simulink model "SDT505SimpleMotorModelBatteryModule220119"  (R2022b)
settings: Solver=VariableStepAuto  StartTime=0.0  StopTime=10.0  RelTol=1e-3
settings Model: Creator=mjbou  LastModifiedBy=mjbou
settings SolverCC: AlgebraicLoopSolver=TrustRegion
settings DebuggingCC: UnconnectedInputMsg=warning  UnconnectedOutputMsg=warning  UnconnectedLineMsg=warning  SFMachineParentedDataDiag=warning
settings ModelReferenceCC: EnableRefExpFcnMdlSchedulingChecks=on

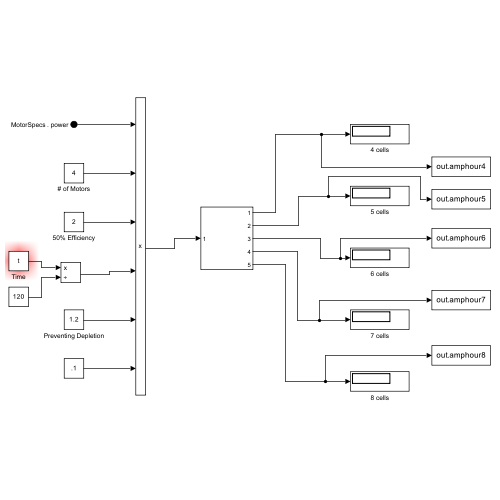
[thumbnail: Simulink's stored preview of the top-level diagram]
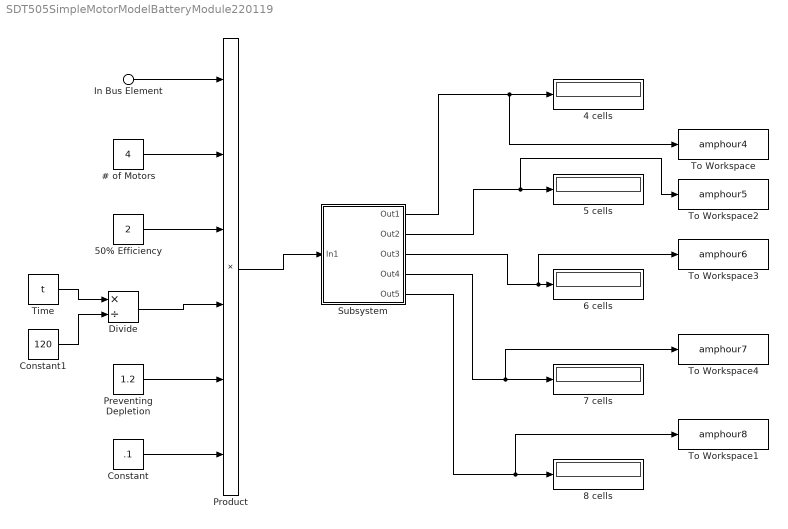
== system SDT505SimpleMotorModelBatteryModule220119 ==
  In Bus Element : Inport  PortName=MotorSpecs  Element=power
  # of Motors : Constant  Value=4
  4 cells : Display
  5 cells : Display
  50% Efficiency : Constant  Value=2
  6 cells : Display
  7 cells : Display
  8 cells : Display
  Constant : Constant  Value=.1
  Constant1 : Constant  Value=120
  Divide : Product  Inputs=*/
  Preventing Depletion : Constant  Value=1.2
  Product : Product  Inputs=6
  Subsystem : Subsystem
  Time : Constant  Value=t
  To Workspace : ToWorkspace  VariableName=amphour4  SaveFormat=Timeseries  SampleTime=-1
  To Workspace1 : ToWorkspace  VariableName=amphour8  SaveFormat=Timeseries  SampleTime=-1
  To Workspace2 : ToWorkspace  VariableName=amphour5  SaveFormat=Timeseries  SampleTime=-1
  To Workspace3 : ToWorkspace  VariableName=amphour6  SaveFormat=Timeseries  SampleTime=-1
  To Workspace4 : ToWorkspace  VariableName=amphour7  SaveFormat=Timeseries  SampleTime=-1
  wires:
  Preventing Depletion/1 -> Product/5
  Product/1 -> Subsystem/1(In1)
  Subsystem/1(Out1) -> To Workspace/1, 4 cells/1
  Subsystem/2(Out2) -> To Workspace2/1, 5 cells/1
  Subsystem/3(Out3) -> To Workspace3/1, 6 cells/1
  Subsystem/4(Out4) -> To Workspace4/1, 7 cells/1
  Subsystem/5(Out5) -> To Workspace1/1, 8 cells/1
  In Bus Element/1 -> Product/1
  Divide/1 -> Product/4
  Time/1 -> Divide/1
  Constant1/1 -> Divide/2
  # of Motors/1 -> Product/2
  50% Efficiency/1 -> Product/3
  Constant/1 -> Product/6

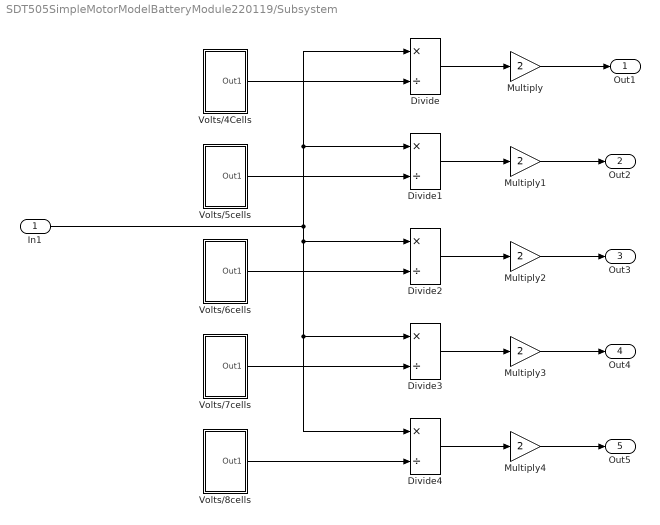
== system SDT505SimpleMotorModelBatteryModule220119/Subsystem ==
  In1 : Inport
  Divide{,1..4} (5 alike) : Product  Inputs=*/
  Multiply{,1..4} (5 alike) : Gain  Gain=2
  Volts/4Cells : Subsystem
  Volts/5cells : Subsystem
  Volts/6cells : Subsystem
  Volts/7cells : Subsystem
  Volts/8cells : Subsystem
  Out1 : Outport
  Out2 : Outport  Port=2
  Out3 : Outport  Port=3
  Out4 : Outport  Port=4
  Out5 : Outport  Port=5
  wires:
  In1/1 -> Divide4/1, Divide3/1, Divide2/1, Divide1/1, Divide/1
  Volts/7cells/1(Out1) -> Divide3/2
  Volts/5cells/1(Out1) -> Divide1/2
  Volts/6cells/1(Out1) -> Divide2/2
  Volts/8cells/1(Out1) -> Divide4/2
  Volts/4Cells/1(Out1) -> Divide/2
  Multiply/1 -> Out1/1
  Divide/1 -> Multiply/1
  Divide1/1 -> Multiply1/1
  Multiply1/1 -> Out2/1
  Divide2/1 -> Multiply2/1
  Multiply2/1 -> Out3/1
  Divide3/1 -> Multiply3/1
  Multiply3/1 -> Out4/1
  Divide4/1 -> Multiply4/1
  Multiply4/1 -> Out5/1

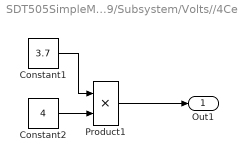
== system SDT505SimpleMotorModelBatteryModule220119/Subsystem/Volts//4Cells ==
  Constant1 : Constant  Value=3.7
  Constant2 : Constant  Value=4
  Product1 : Product
  Out1 : Outport
  wires:
  Constant2/1 -> Product1/2
  Constant1/1 -> Product1/1
  Product1/1 -> Out1/1

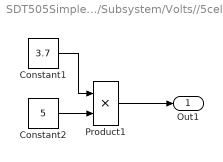
== system SDT505SimpleMotorModelBatteryModule220119/Subsystem/Volts//5cells ==
  Constant1 : Constant  Value=3.7
  Constant2 : Constant  Value=5
  Product1 : Product
  Out1 : Outport
  wires:
  Constant2/1 -> Product1/2
  Constant1/1 -> Product1/1
  Product1/1 -> Out1/1

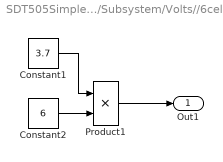
== system SDT505SimpleMotorModelBatteryModule220119/Subsystem/Volts//6cells ==
  Constant1 : Constant  Value=3.7
  Constant2 : Constant  Value=6
  Product1 : Product
  Out1 : Outport
  wires:
  Constant2/1 -> Product1/2
  Constant1/1 -> Product1/1
  Product1/1 -> Out1/1

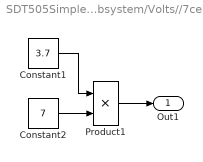
== system SDT505SimpleMotorModelBatteryModule220119/Subsystem/Volts//7cells ==
  Constant1 : Constant  Value=3.7
  Constant2 : Constant  Value=7
  Product1 : Product
  Out1 : Outport
  wires:
  Constant2/1 -> Product1/2
  Constant1/1 -> Product1/1
  Product1/1 -> Out1/1

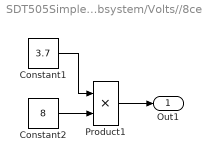
== system SDT505SimpleMotorModelBatteryModule220119/Subsystem/Volts//8cells ==
  Constant1 : Constant  Value=3.7
  Constant2 : Constant  Value=8
  Product1 : Product
  Out1 : Outport
  wires:
  Constant2/1 -> Product1/2
  Constant1/1 -> Product1/1
  Product1/1 -> Out1/1
